simulink model "expe6"  (Simulink 8.3)
settings: Solver=ode45  StartTime=0.0  StopTime=2  RelTol=1e-3
undefined symbols (not defined in the file): A, B, C, D, H
settings Model: Creator=unieerisantos  LastModifiedBy=unieerisantos
settings DataIOCC: SignalLoggingSaveFormat=Dataset
settings DebuggingCC: UnderspecifiedInitializationDetection=Simplified  StateNameClashWarn=none
settings GRTTargetCC: CombineOutputUpdateFcns=on  GRTInterface=off

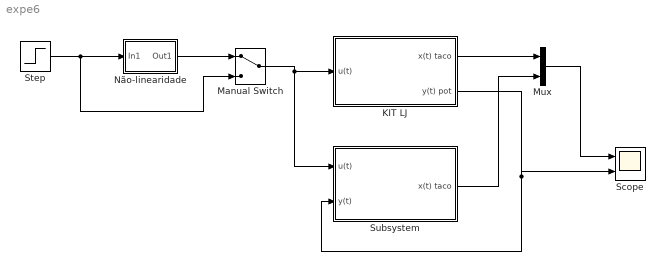
== system expe6 ==
  KIT LJ : Subsystem
  Manual Switch : ManualSwitch
  Mux : Mux  Inputs=2
  "Não-linearidade " : Subsystem
  Scope : Scope  NumInputPorts=2
      settings: YMin=-5~-5  YMax=5~5
  Step : Step  SampleTime=0
  Subsystem : Subsystem
  wires:
  Step/1 -> Manual Switch/2, "Não-linearidade "/1(In1)
  Manual Switch/1 -> Subsystem/1(u(t)), KIT LJ/1(u(t))
  KIT LJ/2(y(t) pot) -> Subsystem/2(y(t)), Scope/2
  "Não-linearidade "/1(Out1) -> Manual Switch/1
  KIT LJ/1(x(t) taco) -> Mux/1
  Subsystem/1(x(t) taco) -> Mux/2
  Mux/1 -> Scope/1

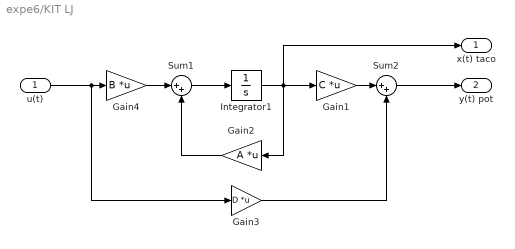
== system expe6/KIT LJ ==
  u(t) : Inport
  Gain1 : Gain  Gain=C  Multiplication=Matrix(K*u)
  Gain2 : Gain  Gain=A  Multiplication=Matrix(K*u)
  Gain3 : Gain  Gain=D  Multiplication=Matrix(K*u)
  Gain4 : Gain  Gain=B  Multiplication=Matrix(K*u)
  Integrator1 : Integrator
  Sum1 : Sum  Inputs=|++
  Sum2 : Sum  Inputs=|++
  x(t) taco : Outport
  y(t) pot : Outport  Port=2
  wires:
  Gain4/1 -> Sum1/1
  Integrator1/1 -> x(t) taco/1, Gain2/1, Gain1/1
  Sum1/1 -> Integrator1/1
  Gain2/1 -> Sum1/2
  Sum2/1 -> y(t) pot/1
  Gain1/1 -> Sum2/1
  Gain3/1 -> Sum2/2
  u(t)/1 -> Gain3/1, Gain4/1

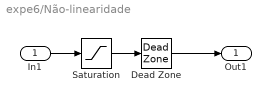
== system expe6/Não-linearidade  ==
  In1 : Inport
  Dead Zone : DeadZone  LowerValue=-0.2  UpperValue=0.2  SaturateOnIntegerOverflow=on
  Saturation : Saturate  UpperLimit=5  LowerLimit=-5
  Out1 : Outport
  wires:
  Saturation/1 -> Dead Zone/1
  Dead Zone/1 -> Out1/1
  In1/1 -> Saturation/1

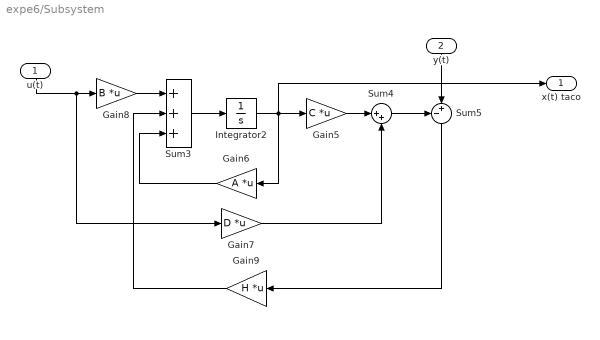
== system expe6/Subsystem ==
  u(t) : Inport
  y(t) : Inport  Port=2
  Gain5 : Gain  Gain=C  Multiplication=Matrix(K*u)
  Gain6 : Gain  Gain=A  Multiplication=Matrix(K*u)
  Gain7 : Gain  Gain=D  Multiplication=Matrix(K*u)
  Gain8 : Gain  Gain=B  Multiplication=Matrix(K*u)
  Gain9 : Gain  Gain=H  Multiplication=Matrix(K*u)
  Integrator2 : Integrator
  Sum3 : Sum  Inputs=+++
  Sum4 : Sum  Inputs=|++
  Sum5 : Sum  Inputs=-+|
  x(t) taco : Outport
  wires:
  Gain6/1 -> Sum3/3
  Gain9/1 -> Sum3/2
  Integrator2/1 -> x(t) taco/1, Gain5/1, Gain6/1
  Sum4/1 -> Sum5/1
  Sum5/1 -> Gain9/1
  Sum3/1 -> Integrator2/1
  Gain7/1 -> Sum4/2
  Gain5/1 -> Sum4/1
  Gain8/1 -> Sum3/1
  y(t)/1 -> Sum5/2
  u(t)/1 -> Gain8/1, Gain7/1
